simulink library "HEV_Electrical_Lib"  (R2019b)
settings: Solver=ode23t  StartTime=0.0  StopTime=10.0  MaxStep=1e-3  RelTol=1e-3
undefined symbols (not defined in the file): DiscIntNeverNeededParam, HEV_Param, magnitude, Ts
libraries: fl_lib x83, powerlib x61, nesl_utility x32, simulink_extras x8, simulink x6, electricdrivelib x4, HEV_Battery_Det_Lib x2, powerlib_extras x2, ee_lib x2, HEV_Battery_Lib x1
(part 2 of 4)

== system HEV_Electrical_Lib/System Level/Speed Sensor SyncGen ==
  MRRef : fl_lib/Mechanical/Rotational Elements/Mechanical Rotational Reference
  PS-Simulink Converter : nesl_utility/PS-Simulink Converter  PhysicalDomain=network_engine_domain  SubClassName=ps_output  LeftPortType=input  RightPortType=output  PseudoPeriodic=off  Frequencies=[]  Unit=rpm  AffineConversion=off
  Rotational Motion Sensor : fl_lib/Mechanical/Mechanical Sensors/Ideal Rotational Motion Sensor  offset=0 rad
  Sh : PMIOPort  Side=Left
  Sh1 : PMIOPort  Port=2  Side=Right
  tag scope: Gen_RPM_SYS=global
  wires:
  PS-Simulink Converter/1 -> [Gen_RPM_SYS]  "Gen_RPM"
  connections:
  Rotational Motion Sensor/RConn1 -- MRRef/LConn1
  PS-Simulink Converter/LConn1 -- Rotational Motion Sensor/RConn2
  Sh1/RConn1 -- Sh/RConn1 -- Rotational Motion Sensor/LConn1

== system HEV_Electrical_Lib/System Level/Speed Sensor SyncMot ==
  MRRef : fl_lib/Mechanical/Rotational Elements/Mechanical Rotational Reference
  PS-Simulink Converter : nesl_utility/PS-Simulink Converter  PhysicalDomain=network_engine_domain  SubClassName=ps_output  LeftPortType=input  RightPortType=output  PseudoPeriodic=off  Frequencies=[]  Unit=rpm  AffineConversion=off
  Rotational Motion Sensor : fl_lib/Mechanical/Mechanical Sensors/Ideal Rotational Motion Sensor  offset=0 rad
  Sh : PMIOPort  Side=Left
  Sh1 : PMIOPort  Port=2  Side=Right
  tag scope: Mot_RPM_SYS=global
  wires:
  PS-Simulink Converter/1 -> [Mot_RPM_SYS]  "Mot_RPM"
  connections:
  Rotational Motion Sensor/RConn1 -- MRRef/LConn1
  Sh1/RConn1 -- Rotational Motion Sensor/LConn1 -- Sh/RConn1
  PS-Simulink Converter/LConn1 -- Rotational Motion Sensor/RConn2

== system HEV_Electrical_Lib/System Level/Synchronous Generator & Drive ==
  note: Note that the generator can turn backwards - this happens when accelerating from rest. The
      | generator also acts as a starter for the engine. If the engine is running, then the generator
      | controller is used to manage battery charging using torque-control mode, otherwise the
      | generator controller controls generator speed.
  TReq : Inport
  GF : Subsystem
      mask Display: disp('GF')
  Inertia : fl_lib/Mechanical/Rotational Elements/Inertia  inertia=HEV_Param.Generator.Shaft_Inertia kg*m^2  w_specify=on  w_priority=High  w=0 rad/s  w_nominal_specify=off  w_nominal_unit=rad/s  w_nominal_value=1  t_specify=off  t_priority=High  t=0 N*m  t_nominal_specify=off  t_nominal_unit=N*m  t_nominal_value=1
  MRRef : fl_lib/Mechanical/Rotational Elements/Mechanical Rotational Reference
  PS Terminator : Subsystem
      mask Display:
      | plot([0 0.9],[0.5 0.5]);
      | plot([0.5 0.9],[0.3 0.3]);
      | plot([0.5 0.9],[0.7 0.7]);
      | plot([0.9 0.9],[0.7 0.3]);
  Power Sensor : Subsystem
      mask Display: disp('S')
  Power and Torque Sensor : Subsystem
      mask Display: disp('S')
  Servomotor : ee_lib/Electromechanical/Permanent Magnet/Simplified PMSM Drive  torque_speed_param=1  w_t=HEV_Param.Generator.TorqSpdLUT.SpeedRPM rpm  T_t=HEV_Param.Generator.TorqSpdLUT.TorqueNm N*m  torque_max=0.1 N*m  power_max=30 W  Tc=HEV_Param.Generator.TorqueControl_TimeConst s  losses_param=1  eff=90  w_eff=2000 rpm  T_eff=200 N*m  Piron=0 W  Pbase=HEV_Param.Generator.TorqIndep_Elec_Loss W  w_eff_vec=[-8000 -4000 0 4000 8000] rpm  T_eff_vec=[0 0.03 0.06 0.09] N*m  v_eff_vec=[100, 250, 400] V  losses_mat=[1.49 1.67 2.21 3.10; 0.42 0.69 1.14 2.03; 0.06 0.24 0.78 1.68; 0.42 0.69 1.14 2.03; 1.49 1.67 2.21 3.10] W  efficiency_mat=[95 95 95 95; 95 95 95 95; 95 95 95 95; 95 95 95 95; 95 95 95 95]  losses_mat_3D=ones(5, 4, 3) W  efficiency_mat_3D=95 * ones(5, 4, 3)  Res=HEV_Param.Generator.Series_Resistance Ohm  J=0 kg*m^2  lam=HEV_Param.Generator.Damping N*m/(rad/s)  speed0=0 rpm  faulted_specify=off  faulted_priority=None  faulted=0  faulted_nominal_specify=off  faulted_nominal_unit=1  faulted_nominal_value=1  alpha=3.93e-3 1/K  Tmeas=25 degC  Tmeas2=125 degC  losses_mat_T2=[1.49, 1.74, 2.49, 3.74; .42, .67, 1.42, 2.67; .06, .31, 1.06, 2.31; .42, .67, 1.42, 2.67; 1.49, 1.74, 2.49, 3.74] W  efficiency_mat_T2=[95, 95, 95, 95; 95, 95, 95, 95; 95, 95, 95, 95; 95, 95, 95, 95; 95, 95, 95, 95]  losses_mat_3D_T2=ones(5, 4, 3) W  efficiency_mat_3D_T2=95 * ones(5, 4, 3)  thermal_mass=100 J/K  initial_temperature=25 degC  fault_condition=1  fault_threshold=0.5
      settings: SourceProductName=Simscape Electrical  SourceProductBaseCode=PS  InternalSimscapePortConfiguration="{\"Bottom\":[],\"Left\":[{\"id\":\"Vp\",\"label\":\"+\",\"type\":\"foundation.electrical.electrical\"},{\"id\":\"Tr\",\"label\":\"Tr\",\"type\":\"input\"},{\"id\":\"R\",\"label\":\"R\",\"type\":\"foundation.mechanical.rotational.rotational\"}],\"Right\":[{\"id\":\"Vm\",\"label\":\"-\",\"type\":\"foundation.electrical.electrical\"},{\"id\":\"Omega\",\"label\":\"w\",\"type\":\"output\"},{\"id\":\"C\",\"label\":\"C\",\"type\":\"foundation.mechanical.rotational.rotational\"}],\"Top\":[]}"
  Vcc : PMIOPort  Side=Right
  Gnd : PMIOPort  Port=2  Side=Right
  Shaft : PMIOPort  Port=3  Side=Right
  wires:
  TReq/1 -> GF/1(In1)
  connections:
  MRRef/LConn1 -- Servomotor/RConn3
  Power and Torque Sensor/LConn1 -- Servomotor/LConn3
  PS Terminator/LConn1 -- Servomotor/RConn2
  GF/RConn1 -- Servomotor/LConn2
  Power Sensor/RConn1 -- Servomotor/LConn1
  Vcc/RConn1 -- Power Sensor/LConn1
  Gnd/RConn1 -- Servomotor/RConn1 -- Power Sensor/LConn2
  Power and Torque Sensor/RConn1 -- Inertia/LConn1 -- Shaft/RConn1

== system HEV_Electrical_Lib/System Level/Synchronous Motor & Drive ==
  TReq : Inport
  GF : Subsystem
      mask Display: disp('GF')
  Inertia : fl_lib/Mechanical/Rotational Elements/Inertia  inertia=HEV_Param.Motor.Shaft_Inertia kg*m^2  w_specify=on  w_priority=High  w=0 rad/s  w_nominal_specify=off  w_nominal_unit=rad/s  w_nominal_value=1  t_specify=off  t_priority=High  t=0 N*m  t_nominal_specify=off  t_nominal_unit=N*m  t_nominal_value=1
  MRRef : fl_lib/Mechanical/Rotational Elements/Mechanical Rotational Reference
  PS Terminator1 : Subsystem
      mask Display:
      | plot([0 0.9],[0.5 0.5]);
      | plot([0.5 0.9],[0.3 0.3]);
      | plot([0.5 0.9],[0.7 0.7]);
      | plot([0.9 0.9],[0.7 0.3]);
  Power Sensor : Subsystem
      mask Display: disp('S')
  Power and Torque Sensor : Subsystem
      mask Display: disp('S')
  Servomotor : ee_lib/Electromechanical/Permanent Magnet/Simplified PMSM Drive  torque_speed_param=1  w_t=HEV_Param.Motor.TorqSpdLUT.SpeedRPM rpm  T_t=HEV_Param.Motor.TorqSpdLUT.TorqueNm N*m  torque_max=0.1 N*m  power_max=30 W  Tc=HEV_Param.Motor.TorqueControl_TimeConst s  losses_param=1  eff=HEV_Param.Motor.Efficiency  w_eff=2000 rpm  T_eff=200 N*m  Piron=0 W  Pbase=0 W  w_eff_vec=[-8000 -4000 0 4000 8000] rpm  T_eff_vec=[0 0.03 0.06 0.09] N*m  v_eff_vec=[100, 250, 400] V  losses_mat=[1.49 1.67 2.21 3.10; 0.42 0.69 1.14 2.03; 0.06 0.24 0.78 1.68; 0.42 0.69 1.14 2.03; 1.49 1.67 2.21 3.10] W  efficiency_mat=[95 95 95 95; 95 95 95 95; 95 95 95 95; 95 95 95 95; 95 95 95 95]  losses_mat_3D=ones(5, 4, 3) W  efficiency_mat_3D=95 * ones(5, 4, 3)  Res=HEV_Param.Motor.Series_Resistance Ohm  J=0 kg*m^2  lam=HEV_Param.Motor.Damping N*m/(rad/s)  speed0=0 rpm  faulted_specify=off  faulted_priority=None  faulted=0  faulted_nominal_specify=off  faulted_nominal_unit=1  faulted_nominal_value=1  alpha=3.93e-3 1/K  Tmeas=25 degC  Tmeas2=125 degC  losses_mat_T2=[1.49, 1.74, 2.49, 3.74; .42, .67, 1.42, 2.67; .06, .31, 1.06, 2.31; .42, .67, 1.42, 2.67; 1.49, 1.74, 2.49, 3.74] W  efficiency_mat_T2=[95, 95, 95, 95; 95, 95, 95, 95; 95, 95, 95, 95; 95, 95, 95, 95; 95, 95, 95, 95]  losses_mat_3D_T2=ones(5, 4, 3) W  efficiency_mat_3D_T2=95 * ones(5, 4, 3)  thermal_mass=100 J/K  initial_temperature=25 degC  fault_condition=1  fault_threshold=0.5
      settings: SourceProductName=Simscape Electrical  SourceProductBaseCode=PS  InternalSimscapePortConfiguration="{\"Bottom\":[],\"Left\":[{\"id\":\"Vp\",\"label\":\"+\",\"type\":\"foundation.electrical.electrical\"},{\"id\":\"Tr\",\"label\":\"Tr\",\"type\":\"input\"},{\"id\":\"R\",\"label\":\"R\",\"type\":\"foundation.mechanical.rotational.rotational\"}],\"Right\":[{\"id\":\"Vm\",\"label\":\"-\",\"type\":\"foundation.electrical.electrical\"},{\"id\":\"Omega\",\"label\":\"w\",\"type\":\"output\"},{\"id\":\"C\",\"label\":\"C\",\"type\":\"foundation.mechanical.rotational.rotational\"}],\"Top\":[]}"
  Vcc : PMIOPort  Side=Right
  Gnd : PMIOPort  Port=2  Side=Right
  Shaft : PMIOPort  Port=3  Side=Right
  wires:
  TReq/1 -> GF/1(In1)
  connections:
  Servomotor/RConn3 -- MRRef/LConn1
  Power and Torque Sensor/LConn1 -- Servomotor/LConn3
  GF/RConn1 -- Servomotor/LConn2
  Power Sensor/RConn1 -- Servomotor/LConn1
  Vcc/RConn1 -- Power Sensor/LConn1
  Servomotor/RConn1 -- Gnd/RConn1 -- Power Sensor/LConn2
  PS Terminator1/LConn1 -- Servomotor/RConn2
  Inertia/LConn1 -- Power and Torque Sensor/RConn1 -- Shaft/RConn1

== system HEV_Electrical_Lib/System Level/Voltage Sensor ==
  PS-Simulink Converter : nesl_utility/PS-Simulink Converter  PhysicalDomain=network_engine_domain  SubClassName=ps_output  LeftPortType=input  RightPortType=output  PseudoPeriodic=off  Frequencies=[]  Unit=V  AffineConversion=off
  Voltage Sensor : fl_lib/Electrical/Electrical Sensors/Voltage Sensor
  + : PMIOPort  Side=Left
  - : PMIOPort  Port=2  Side=Right
  tag scope: DC_Bus_SYS=global
  wires:
  PS-Simulink Converter/1 -> [DC_Bus_SYS]
  connections:
  -/RConn1 -- Voltage Sensor/RConn2
  +/RConn1 -- Voltage Sensor/LConn1
  Voltage Sensor/RConn1 -- PS-Simulink Converter/LConn1

== system HEV_Electrical_Lib/Detailed/DC//DC Converter/PWM ==
  Ref. : Inport
  Data Type Conversion : DataTypeConversion  SaturateOnIntegerOverflow=on  RndMeth=Zero
  Data Type Conversion1 : DataTypeConversion  SaturateOnIntegerOverflow=on  RndMeth=Zero
  Mux : Mux  Inputs=2
  NOT : Logic  Operator=NOT  Inputs=1  AllPortsSameDT=off  OutDataTypeStr=uint(8)
  Rate Transition : RateTransition
  Relational Operator : RelationalOperator  Operator=>  RndMeth=Nearest
  Sawtooth generator : Subsystem
  Thermal Model : Subsystem
  Zero-Order Hold : ZeroOrderHold  SampleTime=Ts
  Pulses : Outport  VectorParamsAs1DForOutWhenUnconnected=off
  wires:
  NOT/1 -> Mux/2
  Rate Transition/1 -> Zero-Order Hold/1
  Relational Operator/1 -> Data Type Conversion/1
  Data Type Conversion/1 -> Mux/1, NOT/1
  Zero-Order Hold/1 -> Relational Operator/1
  Sawtooth generator/1(Out) -> Relational Operator/2
  Ref./1 -> Rate Transition/1, Thermal Model/1(IBus)
  Mux/1 -> Data Type Conversion1/1
  Data Type Conversion1/1 -> Pulses/1

== system HEV_Electrical_Lib/Detailed/DC//DC Converter/Voltage Controller ==
  Uref : Inport
  UBus : Inport  Port=2
  Clock1 : Clock
  Compare To Constant1 : simulink/Logic and Bit Operations/Compare To Constant  relop=>  const=0.01  OutDataTypeStr=uint8  ZeroCross=off
  Ctrl sat. : Saturate  UpperLimit=0.95  LowerLimit=-0.95
  Discrete-Time Integrator : DiscreteIntegrator  IntegratorMethod=Integration: Trapezoidal  SampleTime=Ts  LimitOutput=on  UpperSaturationLimit=1  LowerSaturationLimit=-1  ICPrevOutput=DiscIntNeverNeededParam  ICPrevScaledInput=DiscIntNeverNeededParam
  Integral gain : Gain  Gain=Ki  SaturateOnIntegerOverflow=on  OutDataTypeStr=Inherit: Same as input  ParamDataTypeStr=Inherit: Same as input
  Product1 : Product  RndMeth=Zero
  Proportional gain : Gain  Gain=Kp  SaturateOnIntegerOverflow=on  OutDataTypeStr=Inherit: Same as input  ParamDataTypeStr=Inherit: Same as input
  Sum1 : Sum  Inputs=+-  SaturateOnIntegerOverflow=on  InputSameDT=on  OutDataTypeStr=Inherit: Same as first input
  Sum2 : Sum  SaturateOnIntegerOverflow=on  InputSameDT=on  OutDataTypeStr=Inherit: Same as first input
  Transfer Fcn : TransferFcn  Denominator=[.0001 1]
  Zero-Order Hold1 : ZeroOrderHold  SampleTime=Ts
  Ec : Outport  InitialOutput=0  VectorParamsAs1DForOutWhenUnconnected=off
  wires:
  Sum2/1 -> Ctrl sat./1
  Discrete-Time Integrator/1 -> Sum2/2
  UBus/1 -> Zero-Order Hold1/1
  Integral gain/1 -> Discrete-Time Integrator/1
  Proportional gain/1 -> Sum2/1
  Ctrl sat./1 -> Ec/1
  Sum1/1 -> Product1/1
  Clock1/1 -> Compare To Constant1/1
  Compare To Constant1/1 -> Product1/2
  Product1/1 -> Integral gain/1, Proportional gain/1
  Zero-Order Hold1/1 -> Transfer Fcn/1
  Transfer Fcn/1 -> Sum1/1
  Uref/1 -> Sum1/2

== system HEV_Electrical_Lib/Detailed/Synchronous Generator & Drive/GF ==
  In1 : Inport
  Out1 : Outport  VectorParamsAs1DForOutWhenUnconnected=off
  tag scope: Gen_TReq_SYS=global
  wires:
  In1/1 -> Out1/1, [Gen_TReq_SYS]

== system HEV_Electrical_Lib/Detailed/Synchronous Generator & Drive/Mux ==
  gates : Inport
  m : Inport  Port=2
  Terminator : Terminator
  g : Outport  VectorParamsAs1DForOutWhenUnconnected=off
  wires:
  gates/1 -> g/1
  m/1 -> Terminator/1

== system HEV_Electrical_Lib/Detailed/Synchronous Generator & Drive/Subsystem ==
  In : Inport
  "+ -> -1" : Gain  Gain=30/pi
  Bus Selector : BusSelector  OutputSignals=Stator current is_a (A),Rotor speed wm (rad/s),Electromagnetic torque Te (N*m)
  Mux1 : Mux  Inputs=2
  Mux2 : Mux  Inputs=3
  Out : Outport  VectorParamsAs1DForOutWhenUnconnected=off
  tag scope: GeneratorDrive=global
  wires:
  In/1 -> Bus Selector/1, Out/1
  "+ -> -1"/1 -> Mux2/2
  [Gen_TReq_SYS] -> Mux1/2
  Bus Selector/2 -> "+ -> -1"/1  "<Rotor speed wm (rad/s)>"
  Bus Selector/3 -> Mux1/1  "<Electromagnetic torque Te (N*m)>"
  Mux1/1 -> Mux2/3
  Bus Selector/1 -> Mux2/1  "<Stator current is_a (A)>"
  Mux2/1 -> [GeneratorDrive]

== system HEV_Electrical_Lib/Detailed/Synchronous Generator & Drive/Subsystem1 ==
  Sig : Inport
  Bus Selector : BusSelector  OutputSignals=Electromagnetic torque Te (N*m)
  Ideal Rotational Motion Sensor : fl_lib/Mechanical/Mechanical Sensors/Ideal Rotational Motion Sensor  offset=0 rad
  Ideal Torque Source : fl_lib/Mechanical/Mechanical Sources/Ideal Torque Source
  Mechanical Rotational Reference : fl_lib/Mechanical/Rotational Elements/Mechanical Rotational Reference
  Mechanical Rotational Reference1 : fl_lib/Mechanical/Rotational Elements/Mechanical Rotational Reference
  PS-Simulink Converter : nesl_utility/PS-Simulink Converter  PhysicalDomain=network_engine_domain  SubClassName=ps_output  LeftPortType=input  RightPortType=output  PseudoPeriodic=off  Frequencies=[]  Unit=rad/s  AffineConversion=off
  Simulink-PS Converter : nesl_utility/Simulink-PS Converter  PhysicalDomain=network_engine_domain  SubClassName=ps_input  LeftPortType=input  RightPortType=output  PseudoPeriodic=off  Frequencies=[]  NoiseDistribution=none  NoiseParameters=[]  Unit=1  AffineConversion=off  FilteringAndDerivatives=zero  SimscapeFilterOrder=1  InputFilterTimeConstant=0.005  UdotUserProvided=0
  Sh : PMIOPort  Side=Right
  Spd : Outport  VectorParamsAs1DForOutWhenUnconnected=off
  wires:
  Bus Selector/1 -> Simulink-PS Converter/1  "<Electromagnetic torque Te (N*m)>"
  Sig/1 -> Bus Selector/1
  PS-Simulink Converter/1 -> Spd/1
  connections:
  Mechanical Rotational Reference/LConn1 -- Ideal Rotational Motion Sensor/RConn1
  Mechanical Rotational Reference1/LConn1 -- Ideal Torque Source/RConn2
  Ideal Torque Source/LConn1 -- Sh/RConn1 -- Ideal Rotational Motion Sensor/LConn1
  PS-Simulink Converter/LConn1 -- Ideal Rotational Motion Sensor/RConn2
  Simulink-PS Converter/RConn1 -- Ideal Torque Source/RConn1

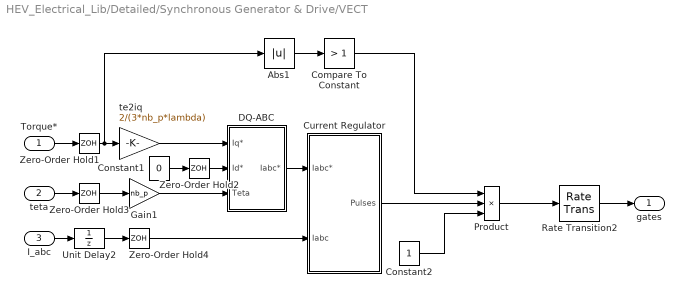
== system HEV_Electrical_Lib/Detailed/Synchronous Generator & Drive/VECT ==
  Torque* : Inport
  teta : Inport  Port=2
  I_abc : Inport  Port=3
  Abs1 : Abs
  Compare To Constant : simulink/Logic and Bit Operations/Compare To Constant  relop=>  const=1  OutDataTypeStr=uint8
  Constant1 : Constant  Value=0
  Constant2 : Constant
  Current Regulator : Subsystem
  DQ-ABC : Subsystem
  Gain1 : Gain  Gain=nb_p  SaturateOnIntegerOverflow=on  OutDataTypeStr=Inherit: Same as input  ParamDataTypeStr=Inherit: Same as input
  Product : Product  Inputs=3  RndMeth=Zero
  Rate Transition2 : RateTransition
  Unit Delay2 : UnitDelay  SampleTime=-1  HasFrameUpgradeWarning=on
  Zero-Order Hold{1..4} (4 alike) : ZeroOrderHold  SampleTime=Ts_vect
  te2iq : Gain  Gain=2/(3*nb_p*lambda)  SaturateOnIntegerOverflow=on  OutDataTypeStr=Inherit: Same as input  ParamDataTypeStr=Inherit: Same as input
  gates : Outport  VectorParamsAs1DForOutWhenUnconnected=off
  wires:
  Compare To Constant/1 -> Product/1
  Abs1/1 -> Compare To Constant/1
  Constant2/1 -> Product/3
  I_abc/1 -> Unit Delay2/1
  DQ-ABC/1(Iabc*) -> Current Regulator/1(Iabc*)
  Gain1/1 -> DQ-ABC/3(Teta)
  Constant1/1 -> Zero-Order Hold2/1
  Torque*/1 -> Zero-Order Hold1/1
  Zero-Order Hold3/1 -> Gain1/1
  teta/1 -> Zero-Order Hold3/1
  Current Regulator/1(Pulses) -> Product/2
  Zero-Order Hold1/1 -> Abs1/1, te2iq/1
  Zero-Order Hold4/1 -> Current Regulator/2(Iabc)
  Zero-Order Hold2/1 -> DQ-ABC/2("Id* ")
  Rate Transition2/1 -> gates/1
  Product/1 -> Rate Transition2/1
  te2iq/1 -> DQ-ABC/1("Iq* ")
  Unit Delay2/1 -> Zero-Order Hold4/1

== system HEV_Electrical_Lib/Detailed/Synchronous Motor & Drive/GF ==
  In1 : Inport
  Out1 : Outport  VectorParamsAs1DForOutWhenUnconnected=off
  tag scope: Mot_TReq_SYS=global
  wires:
  In1/1 -> Out1/1, [Mot_TReq_SYS]

== system HEV_Electrical_Lib/Detailed/Synchronous Motor & Drive/Mux ==
  gates : Inport
  m : Inport  Port=2
  Terminator : Terminator
  g : Outport  VectorParamsAs1DForOutWhenUnconnected=off
  wires:
  m/1 -> Terminator/1
  gates/1 -> g/1

== system HEV_Electrical_Lib/Detailed/Synchronous Motor & Drive/Subsystem ==
  In : Inport
  "+ -> -1" : Gain  Gain=30/pi
  Bus Selector : BusSelector  OutputSignals=Stator current is_a (A),Rotor speed wm (rad/s),Electromagnetic torque Te (N*m)
  Mux1 : Mux  Inputs=2
  Mux2 : Mux  Inputs=3
  Out : Outport  VectorParamsAs1DForOutWhenUnconnected=off
  tag scope: MotorDrive=global
  wires:
  In/1 -> Bus Selector/1, Out/1
  "+ -> -1"/1 -> Mux2/2
  [Mot_TReq_SYS] -> Mux1/2
  Bus Selector/2 -> "+ -> -1"/1  "<Rotor speed wm (rad/s)>"
  Bus Selector/3 -> Mux1/1  "<Electromagnetic torque Te (N*m)>"
  Mux1/1 -> Mux2/3
  Bus Selector/1 -> Mux2/1  "<Stator current is_a (A)>"
  Mux2/1 -> [MotorDrive]

== system HEV_Electrical_Lib/Detailed/Synchronous Motor & Drive/Subsystem1 ==
  Sig : Inport
  Bus Selector : BusSelector  OutputSignals=Electromagnetic torque Te (N*m)
  Ideal Rotational Motion Sensor : fl_lib/Mechanical/Mechanical Sensors/Ideal Rotational Motion Sensor  offset=0 rad
  Ideal Torque Source : fl_lib/Mechanical/Mechanical Sources/Ideal Torque Source
  Mechanical Rotational Reference : fl_lib/Mechanical/Rotational Elements/Mechanical Rotational Reference
  Mechanical Rotational Reference1 : fl_lib/Mechanical/Rotational Elements/Mechanical Rotational Reference
  PS-Simulink Converter : nesl_utility/PS-Simulink Converter  PhysicalDomain=network_engine_domain  SubClassName=ps_output  LeftPortType=input  RightPortType=output  PseudoPeriodic=off  Frequencies=[]  Unit=rad/s  AffineConversion=off
  Simulink-PS Converter : nesl_utility/Simulink-PS Converter  PhysicalDomain=network_engine_domain  SubClassName=ps_input  LeftPortType=input  RightPortType=output  PseudoPeriodic=off  Frequencies=[]  NoiseDistribution=none  NoiseParameters=[]  Unit=1  AffineConversion=off  FilteringAndDerivatives=zero  SimscapeFilterOrder=1  InputFilterTimeConstant=0.005  UdotUserProvided=0
  Sh : PMIOPort  Side=Right
  Spd : Outport  VectorParamsAs1DForOutWhenUnconnected=off
  wires:
  PS-Simulink Converter/1 -> Spd/1
  Sig/1 -> Bus Selector/1
  Bus Selector/1 -> Simulink-PS Converter/1  "<Electromagnetic torque Te (N*m)>"
  connections:
  Simulink-PS Converter/RConn1 -- Ideal Torque Source/RConn1
  PS-Simulink Converter/LConn1 -- Ideal Rotational Motion Sensor/RConn2
  Ideal Rotational Motion Sensor/LConn1 -- Sh/RConn1 -- Ideal Torque Source/LConn1
  Mechanical Rotational Reference1/LConn1 -- Ideal Torque Source/RConn2
  Mechanical Rotational Reference/LConn1 -- Ideal Rotational Motion Sensor/RConn1

== system HEV_Electrical_Lib/Detailed/Synchronous Motor & Drive/Torque limitation ==
  N rad/s : Inport
  Torque : Inport  Port=2
  Abs1 : Abs  SaturateOnIntegerOverflow=on
  Gain : Gain  Gain=-1
  Saturation Dynamic : simulink/Discontinuities/Saturation Dynamic  OutMin=[]  OutMax=[]  OutDataTypeStr=Inherit: Same as second input  OutDataType=sfix(16)  OutScaling=2^-10  DoSatur=off
  Torque vs speed profile : Lookup  InputValues=[0 1200 2000 3000 4000 5000 6000]*pi/30  Table=[400 400 225 150 100 80 70]
  torque : Outport  VectorParamsAs1DForOutWhenUnconnected=off
  wires:
  Gain/1 -> Saturation Dynamic/3
  Torque/1 -> Saturation Dynamic/2
  Saturation Dynamic/1 -> torque/1
  Torque vs speed profile/1 -> Gain/1, Saturation Dynamic/1
  Abs1/1 -> Torque vs speed profile/1
  N rad/s/1 -> Abs1/1

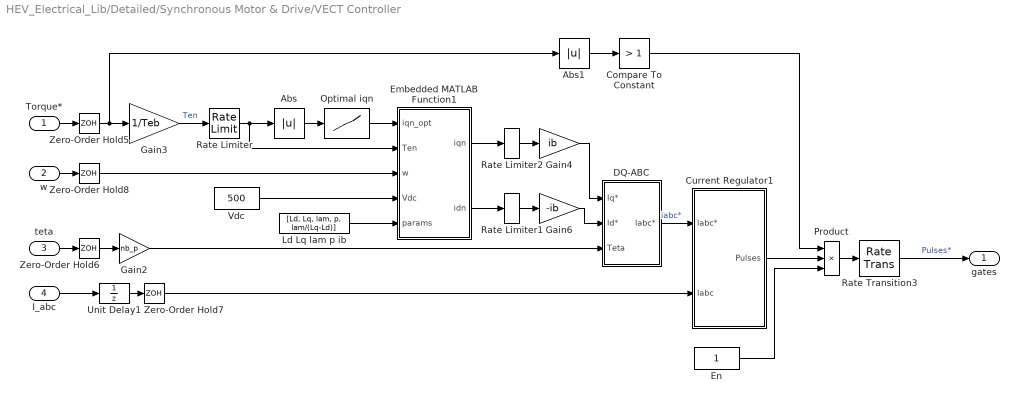
== system HEV_Electrical_Lib/Detailed/Synchronous Motor & Drive/VECT Controller ==
  Torque* : Inport
  w : Inport  Port=2
  teta : Inport  Port=3
  I_abc : Inport  Port=4
  Abs : Abs
  Abs1 : Abs
  Compare To Constant : simulink/Logic and Bit Operations/Compare To Constant  relop=>  const=1  OutDataTypeStr=uint8
  Current Regulator1 : Subsystem
  DQ-ABC : Subsystem
  Embedded MATLAB Function1 : MATLAB Function  TreatAsAtomicUnit=on  SystemSampleTime=Ts_vect
  En : Constant
  Gain2 : Gain  Gain=nb_p  SaturateOnIntegerOverflow=on  OutDataTypeStr=Inherit: Same as input  ParamDataTypeStr=Inherit: Same as input
  Gain3 : Gain  Gain=1/Teb  SaturateOnIntegerOverflow=on  OutDataTypeStr=Inherit: Same as input  ParamDataTypeStr=Inherit: Same as input
  Gain4 : Gain  Gain=ib  SaturateOnIntegerOverflow=on  OutDataTypeStr=Inherit: Same as input  ParamDataTypeStr=Inherit: Same as input
  Gain6 : Gain  Gain=-ib  SaturateOnIntegerOverflow=on  OutDataTypeStr=Inherit: Same as input  ParamDataTypeStr=Inherit: Same as input
  Ld Lq lam p ib : Constant  Value=[Ld, Lq, lam, p, lam/(Lq-Ld)]
  Optimal iqn : Lookup  InputValues=ten  Table=iqn
  Product : Product  Inputs=3  RndMeth=Zero
  Rate Limiter : RateLimiter  RisingSlewLimit=10  FallingSlewLimit=-10  LinearizeAsGain=off
  Rate Limiter1 : RateLimiter  RisingSlewLimit=100  FallingSlewLimit=-100  SampleTimeMode=inherited
  Rate Limiter2 : RateLimiter  RisingSlewLimit=100  FallingSlewLimit=-100  SampleTimeMode=inherited
  Rate Transition3 : RateTransition
  Unit Delay1 : UnitDelay  SampleTime=-1  HasFrameUpgradeWarning=on
  Vdc : Constant  Value=500
  Zero-Order Hold{5..8} (4 alike) : ZeroOrderHold  SampleTime=Ts_vect
  gates : Outport  VectorParamsAs1DForOutWhenUnconnected=off
  wires:
  Abs1/1 -> Compare To Constant/1
  Compare To Constant/1 -> Product/1
  En/1 -> Product/3
  Current Regulator1/1(Pulses) -> Product/2
  Unit Delay1/1 -> Zero-Order Hold7/1
  Zero-Order Hold7/1 -> Current Regulator1/2(Iabc)
  teta/1 -> Zero-Order Hold6/1
  Zero-Order Hold6/1 -> Gain2/1
  Gain2/1 -> DQ-ABC/3(Teta)
  DQ-ABC/1(Iabc*) -> Current Regulator1/1(Iabc*)  "iabc*"
  I_abc/1 -> Unit Delay1/1
  Torque*/1 -> Zero-Order Hold5/1
  Gain4/1 -> DQ-ABC/1("Iq* ")
  Gain6/1 -> DQ-ABC/2("Id* ")
  Zero-Order Hold5/1 -> Abs1/1, Gain3/1
  w/1 -> Zero-Order Hold8/1
  Embedded MATLAB Function1/2(idn) -> Rate Limiter1/1
  Gain3/1 -> Rate Limiter/1  "Ten"
  Zero-Order Hold8/1 -> Embedded MATLAB Function1/3(w)
  Ld Lq lam p ib/1 -> Embedded MATLAB Function1/5(params)
  Embedded MATLAB Function1/1(iqn) -> Rate Limiter2/1
  Optimal iqn/1 -> Embedded MATLAB Function1/1(iqn_opt)
  Abs/1 -> Optimal iqn/1
  Vdc/1 -> Embedded MATLAB Function1/4(Vdc)
  Rate Transition3/1 -> gates/1  "Pulses*"
  Product/1 -> Rate Transition3/1
  Rate Limiter2/1 -> Gain4/1
  Rate Limiter1/1 -> Gain6/1
  Rate Limiter/1 -> Abs/1, Embedded MATLAB Function1/2(Ten)

== system HEV_Electrical_Lib/Mean Value/DC//DC Converter/Boost Converter Average-Values ==
  Duty Cycle : Inport
  Average-value armature voltage : Fcn  Expr=u(1)*u(2)
  Average-value source current : Fcn  Expr=u(1)*u(2)
  Controlled Current Source : powerlib/Electrical Sources/Controlled Current Source  Initialize=on  Source_Type=AC  Amplitude=0  Phase=0  Frequency=0  Measurements=None
      settings: SourceProductName=Simscape Electrical
  Controlled Voltage Source : powerlib/Electrical Sources/Controlled Voltage Source  Initialize=on  Source_Type=AC  Amplitude=0  Phase=0  Frequency=0  Measurements=None
      settings: SourceProductName=Simscape Electrical
  Current Measurement : powerlib/Measurements/Current Measurement  Tag=PoWeRsYsTeMmEaSuReMeNt  PhasorSimulation=off  OutputType=Magnitude  PSBequivalent=0
      settings: SourceProductName=Simscape Electrical
  Mux : Mux  Inputs=2
  Mux1 : Mux  Inputs=2
  Selector : Selector  InputPortWidth=2  IndexOptions=Index vector (dialog)  Indices=[1]  OutputSizes=1
  Thermal Model : Subsystem
  Unit Delay : UnitDelay  SampleTime=Ts  HasFrameUpgradeWarning=on
  Unit Delay1 : UnitDelay  SampleTime=Ts  HasFrameUpgradeWarning=on
  Voltage Measurement1 : powerlib/Measurements/Voltage Measurement  Tag=PoWeRsYsTeMmEaSuReMeNt  PhasorSimulation=off  OutputType=Magnitude  PSBequivalent=0
      settings: SourceProductName=Simscape Electrical
  A : PMIOPort  Side=Right
  + : PMIOPort  Port=2  Side=Left
  - : PMIOPort  Port=3  Side=Left
  wires:
  Unit Delay/1 -> Controlled Voltage Source/1
  Average-value armature voltage/1 -> Unit Delay/1
  Mux/1 -> Average-value armature voltage/1
  Voltage Measurement1/1 -> Mux/2
  Duty Cycle/1 -> Selector/1
  Mux1/1 -> Average-value source current/1
  Current Measurement/1 -> Mux1/2
  Average-value source current/1 -> Unit Delay1/1
  Unit Delay1/1 -> Controlled Current Source/1, Thermal Model/1(IBus)
  Selector/1 -> Mux/1, Mux1/1
  connections:
  Voltage Measurement1/LConn2 -- Controlled Current Source/RConn1 -- -/RConn1 -- Controlled Voltage Source/LConn1
  Controlled Current Source/LConn1 -- Voltage Measurement1/LConn1 -- +/RConn1
  Controlled Voltage Source/RConn1 -- Current Measurement/LConn1
  A/RConn1 -- Current Measurement/RConn1

== system HEV_Electrical_Lib/Mean Value/DC//DC Converter/Current controller DISCRETE3 ==
  Uref : Inport
  UBus : Inport  Port=2
  Clock1 : Clock
  Compare To Constant1 : simulink/Logic and Bit Operations/Compare To Constant  relop=>  const=0.01  OutDataTypeStr=uint8  ZeroCross=off
  Ctrl sat. : Saturate  UpperLimit=0.95  LowerLimit=-0.95
  Discrete-Time Integrator : DiscreteIntegrator  IntegratorMethod=Integration: Trapezoidal  SampleTime=Ts  LimitOutput=on  UpperSaturationLimit=1  LowerSaturationLimit=-1  ICPrevOutput=DiscIntNeverNeededParam  ICPrevScaledInput=DiscIntNeverNeededParam
  Integral gain : Gain  Gain=Ki  SaturateOnIntegerOverflow=on  OutDataTypeStr=Inherit: Same as input  ParamDataTypeStr=Inherit: Same as input
  Product1 : Product  RndMeth=Zero
  Proportional gain : Gain  Gain=Kp  SaturateOnIntegerOverflow=on  OutDataTypeStr=Inherit: Same as input  ParamDataTypeStr=Inherit: Same as input
  Sum1 : Sum  Inputs=+-  SaturateOnIntegerOverflow=on  InputSameDT=on  OutDataTypeStr=Inherit: Same as first input
  Sum2 : Sum  SaturateOnIntegerOverflow=on  InputSameDT=on  OutDataTypeStr=Inherit: Same as first input
  Transfer Fcn : TransferFcn  Denominator=[.0001 1]
  Zero-Order Hold1 : ZeroOrderHold  SampleTime=Ts
  Ec : Outport  InitialOutput=0  VectorParamsAs1DForOutWhenUnconnected=off
  wires:
  Sum2/1 -> Ctrl sat./1
  Discrete-Time Integrator/1 -> Sum2/2
  UBus/1 -> Zero-Order Hold1/1
  Integral gain/1 -> Discrete-Time Integrator/1
  Proportional gain/1 -> Sum2/1
  Ctrl sat./1 -> Ec/1
  Sum1/1 -> Product1/1
  Clock1/1 -> Compare To Constant1/1
  Compare To Constant1/1 -> Product1/2
  Product1/1 -> Integral gain/1, Proportional gain/1
  Zero-Order Hold1/1 -> Transfer Fcn/1
  Transfer Fcn/1 -> Sum1/1
  Uref/1 -> Sum1/2

== system HEV_Electrical_Lib/Mean Value/DC//DC Converter/Duty Cycles ==
  Ec : Inport
  Add : Sum  Inputs=+-
  Bus Creator2 : BusCreator  Inputs=2
  Constant : Constant
  Duty Cycle : Fcn  Expr=0.5*(u[1]+1)
  Unit Delay2 : UnitDelay  InitialCondition=.5  SampleTime=Ts  HasFrameUpgradeWarning=on
  dc : Outport  VectorParamsAs1DForOutWhenUnconnected=off
  wires:
  Bus Creator2/1 -> Unit Delay2/1
  Ec/1 -> Duty Cycle/1
  Constant/1 -> Add/1
  Add/1 -> Bus Creator2/2  "IGBT 2"
  Duty Cycle/1 -> Bus Creator2/1, Add/2  "IGBT I"
  Unit Delay2/1 -> dc/1

== system HEV_Electrical_Lib/Mean Value/Synchronous Generator & Drive/GF ==
  In1 : Inport
  Out1 : Outport  VectorParamsAs1DForOutWhenUnconnected=off
  tag scope: Gen_TReq_SYS=global
  wires:
  In1/1 -> Out1/1, [Gen_TReq_SYS]

== system HEV_Electrical_Lib/Mean Value/Synchronous Generator & Drive/Mux ==
  sig* : Inport
  m : Inport  Port=2
  Bus Creator : BusCreator  Inputs=2
  Ctrl : Outport  VectorParamsAs1DForOutWhenUnconnected=off
  wires:
  Bus Creator/1 -> Ctrl/1
  sig*/1 -> Bus Creator/1  "Signals*"
  m/1 -> Bus Creator/2  "m"

== system HEV_Electrical_Lib/Mean Value/Synchronous Generator & Drive/Subsystem ==
  In : Inport
  "+ -> -1" : Gain  Gain=30/pi
  Bus Selector : BusSelector  OutputSignals=Stator current is_a (A),Rotor speed wm (rad/s),Electromagnetic torque Te (N*m)
  Mux1 : Mux  Inputs=2
  Mux2 : Mux  Inputs=3
  Out : Outport  VectorParamsAs1DForOutWhenUnconnected=off
  tag scope: GeneratorDrive=global
  wires:
  In/1 -> Bus Selector/1, Out/1
  "+ -> -1"/1 -> Mux2/2
  [Gen_TReq_SYS] -> Mux1/2
  Bus Selector/2 -> "+ -> -1"/1  "<Rotor speed wm (rad/s)>"
  Bus Selector/3 -> Mux1/1  "<Electromagnetic torque Te (N*m)>"
  Mux1/1 -> Mux2/3
  Bus Selector/1 -> Mux2/1  "<Stator current is_a (A)>"
  Mux2/1 -> [GeneratorDrive]

== system HEV_Electrical_Lib/Mean Value/Synchronous Generator & Drive/Subsystem1 ==
  Sig : Inport
  Bus Selector : BusSelector  OutputSignals=Electromagnetic torque Te (N*m)
  Ideal Rotational Motion Sensor : fl_lib/Mechanical/Mechanical Sensors/Ideal Rotational Motion Sensor  offset=0 rad
  Ideal Torque Source : fl_lib/Mechanical/Mechanical Sources/Ideal Torque Source
  Mechanical Rotational Reference : fl_lib/Mechanical/Rotational Elements/Mechanical Rotational Reference
  Mechanical Rotational Reference1 : fl_lib/Mechanical/Rotational Elements/Mechanical Rotational Reference
  PS-Simulink Converter : nesl_utility/PS-Simulink Converter  PhysicalDomain=network_engine_domain  SubClassName=ps_output  LeftPortType=input  RightPortType=output  PseudoPeriodic=off  Frequencies=[]  Unit=rad/s  AffineConversion=off
  Simulink-PS Converter : nesl_utility/Simulink-PS Converter  PhysicalDomain=network_engine_domain  SubClassName=ps_input  LeftPortType=input  RightPortType=output  PseudoPeriodic=off  Frequencies=[]  NoiseDistribution=none  NoiseParameters=[]  Unit=1  AffineConversion=off  FilteringAndDerivatives=zero  SimscapeFilterOrder=1  InputFilterTimeConstant=0.005  UdotUserProvided=0
  Sh : PMIOPort  Side=Right
  Spd : Outport  VectorParamsAs1DForOutWhenUnconnected=off
  wires:
  PS-Simulink Converter/1 -> Spd/1
  Sig/1 -> Bus Selector/1
  Bus Selector/1 -> Simulink-PS Converter/1  "<Electromagnetic torque Te (N*m)>"
  connections:
  Simulink-PS Converter/RConn1 -- Ideal Torque Source/RConn1
  PS-Simulink Converter/LConn1 -- Ideal Rotational Motion Sensor/RConn2
  Ideal Rotational Motion Sensor/LConn1 -- Sh/RConn1 -- Ideal Torque Source/LConn1
  Mechanical Rotational Reference1/LConn1 -- Ideal Torque Source/RConn2
  Mechanical Rotational Reference/LConn1 -- Ideal Rotational Motion Sensor/RConn1

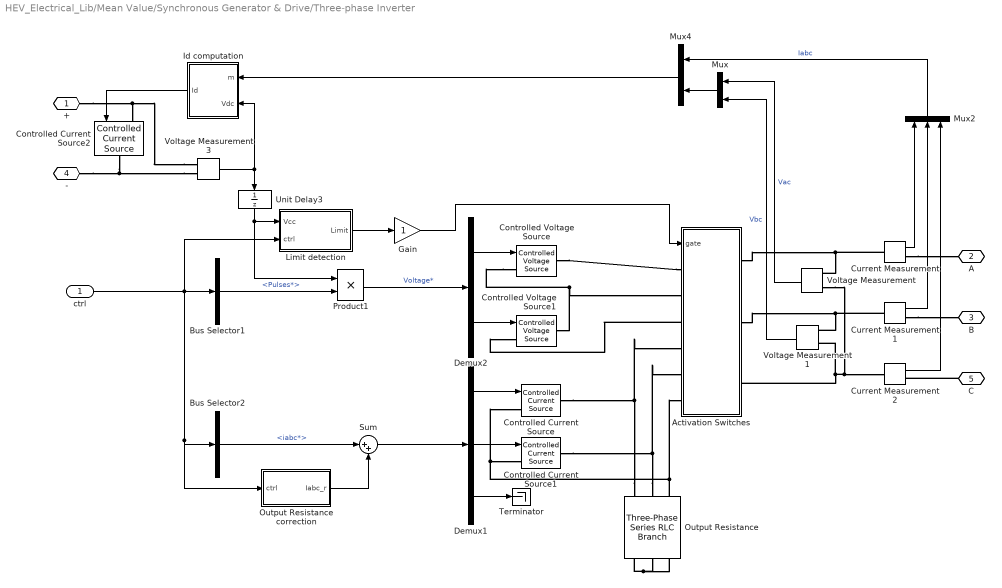
== system HEV_Electrical_Lib/Mean Value/Synchronous Generator & Drive/Three-phase Inverter ==
  ctrl : Inport
  Activation Switches : Subsystem
  Bus Selector1 : BusSelector  OutputSignals=Signals*.Pulses*
  Bus Selector2 : BusSelector  OutputSignals=Signals*.iabc*
  Controlled Current Source : powerlib/Electrical Sources/Controlled Current Source  Initialize=on  Source_Type=AC  Amplitude=0  Phase=0  Frequency=0  Measurements=None
      settings: SourceProductName=Simscape Electrical
  Controlled Current Source1 : powerlib/Electrical Sources/Controlled Current Source  Initialize=on  Source_Type=AC  Amplitude=0  Phase=0  Frequency=0  Measurements=None
      settings: SourceProductName=Simscape Electrical
  Controlled Current Source2 : powerlib/Electrical Sources/Controlled Current Source  Initialize=on  Source_Type=AC  Amplitude=0  Phase=0  Frequency=0  Measurements=None
      settings: SourceProductName=Simscape Electrical
  Controlled Voltage Source : powerlib/Electrical Sources/Controlled Voltage Source  Initialize=on  Source_Type=AC  Amplitude=0  Phase=0  Frequency=0  Measurements=None
      settings: SourceProductName=Simscape Electrical
  Controlled Voltage Source1 : powerlib/Electrical Sources/Controlled Voltage Source  Initialize=on  Source_Type=AC  Amplitude=0  Phase=0  Frequency=0  Measurements=None
      settings: SourceProductName=Simscape Electrical
  Current Measurement : powerlib/Measurements/Current Measurement  PhasorSimulation=off  OutputType=Complex  PSBequivalent=0
      settings: SourceProductName=Simscape Electrical
  Current Measurement1 : powerlib/Measurements/Current Measurement  PhasorSimulation=off  OutputType=Complex  PSBequivalent=0
      settings: SourceProductName=Simscape Electrical
  Current Measurement2 : powerlib/Measurements/Current Measurement  PhasorSimulation=off  OutputType=Complex  PSBequivalent=0
      settings: SourceProductName=Simscape Electrical
  Demux1 : Demux  Outputs=3
  Demux2 : Demux  Outputs=2
  Gain : Gain
  Id computation : Subsystem
  Limit detection : Subsystem
  Mux : Mux  Inputs=2
  Mux2 : Mux  Inputs=3
  Mux4 : Mux  Inputs=2
  Output Resistance : powerlib/Elements/Three-Phase Series RLC Branch  LConnTagsString=A|B|C  RConnTagsString=A|B|C  BranchType=R  Resistance=100*Resistance  Inductance=1e-3  Capacitance=1e-6  Measurements=Branch voltages and currents
      settings: SourceProductName=Simscape Electrical
  Output Resistance correction : Subsystem
  Product1 : Product  RndMeth=Zero
  Sum : Sum  Inputs=|++
  Terminator : Terminator
  Unit Delay3 : UnitDelay  SampleTime=Ts  HasFrameUpgradeWarning=on
  Voltage Measurement : powerlib/Measurements/Voltage Measurement  PhasorSimulation=off  OutputType=Complex  PSBequivalent=0
      settings: SourceProductName=Simscape Electrical
  Voltage Measurement1 : powerlib/Measurements/Voltage Measurement  PhasorSimulation=off  OutputType=Complex  PSBequivalent=0
      settings: SourceProductName=Simscape Electrical
  Voltage Measurement3 : powerlib/Measurements/Voltage Measurement  PhasorSimulation=off  OutputType=Complex  PSBequivalent=0
      settings: SourceProductName=Simscape Electrical
  + : PMIOPort  Side=Right
  A : PMIOPort  Port=2  Side=Left
  B : PMIOPort  Port=3  Side=Left
  - : PMIOPort  Port=4  Side=Right
  C : PMIOPort  Port=5  Side=Left
  wires:
  Current Measurement/1 -> Mux2/1
  Current Measurement1/1 -> Mux2/2
  Voltage Measurement/1 -> Mux/1  "Vac"
  Voltage Measurement1/1 -> Mux/2  "Vbc"
  Mux/1 -> Mux4/2
  Current Measurement2/1 -> Mux2/3
  Mux4/1 -> Id computation/1(m)
  Mux2/1 -> Mux4/1  "Iabc"
  Id computation/1(Id) -> Controlled Current Source2/1
  Voltage Measurement3/1 -> Unit Delay3/1, Id computation/2(Vdc)
  Bus Selector1/1 -> Product1/2  "<Pulses*>"
  Demux1/1 -> Controlled Current Source/1
  Demux1/2 -> Controlled Current Source1/1
  Demux1/3 -> Terminator/1
  Demux2/2 -> Controlled Voltage Source1/1
  Demux2/1 -> Controlled Voltage Source/1
  Bus Selector2/1 -> Sum/1  "<iabc*>"
  Limit detection/1(Limit) -> Gain/1
  Sum/1 -> Demux1/1
  Unit Delay3/1 -> Product1/1, Limit detection/1(Vcc)
  ctrl/1 -> Bus Selector1/1, Limit detection/2(ctrl), Bus Selector2/1, Output Resistance correction/1(ctrl)
  Product1/1 -> Demux2/1  "Voltage*"
  Output Resistance correction/1("Iabc_r ") -> Sum/2
  Gain/1 -> Activation Switches/1(gate)
  connections:
  Voltage Measurement3/LConn1 -- Controlled Current Source2/LConn1 -- +/RConn1
  Voltage Measurement3/LConn2 -- Controlled Current Source2/RConn1 -- -/RConn1
  Activation Switches/LConn6 -- Controlled Current Source/LConn1 -- Controlled Current Source1/LConn1 -- Output Resistance/LConn3
  Output Resistance/RConn3 -- Output Resistance/RConn2 -- Output Resistance/RConn1
  Voltage Measurement/LConn1 -- Activation Switches/RConn1 -- Current Measurement/LConn1
  Output Resistance/LConn1 -- Activation Switches/LConn4 -- Controlled Current Source/RConn1
  Output Resistance/LConn2 -- Activation Switches/LConn5 -- Controlled Current Source1/RConn1
  Voltage Measurement/LConn2 -- Activation Switches/RConn3 -- Voltage Measurement1/LConn2 -- Current Measurement2/LConn1
  Controlled Voltage Source/LConn1 -- Activation Switches/LConn2 -- Controlled Voltage Source1/RConn1
  Voltage Measurement1/LConn1 -- Activation Switches/RConn2 -- Current Measurement1/LConn1
  Current Measurement/RConn1 -- A/RConn1
  Current Measurement1/RConn1 -- B/RConn1
  C/RConn1 -- Current Measurement2/RConn1
  Controlled Voltage Source/RConn1 -- Activation Switches/LConn1
  Activation Switches/LConn3 -- Controlled Voltage Source1/LConn1

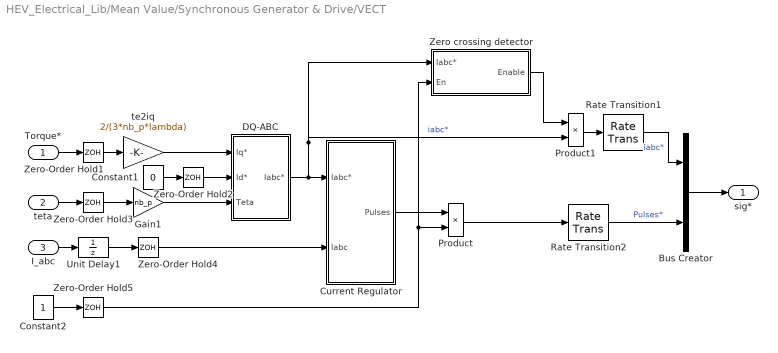
== system HEV_Electrical_Lib/Mean Value/Synchronous Generator & Drive/VECT ==
  Torque* : Inport
  teta : Inport  Port=2
  I_abc : Inport  Port=3
  Bus Creator : BusCreator  Inputs=2
  Constant1 : Constant  Value=0
  Constant2 : Constant
  Current Regulator : Subsystem
  DQ-ABC : Subsystem
  Gain1 : Gain  Gain=nb_p  SaturateOnIntegerOverflow=on  OutDataTypeStr=Inherit: Same as input  ParamDataTypeStr=Inherit: Same as input
  Product : Product  RndMeth=Zero
  Product1 : Product  RndMeth=Zero
  Rate Transition1 : RateTransition
  Rate Transition2 : RateTransition
  Unit Delay1 : UnitDelay  SampleTime=Ts  HasFrameUpgradeWarning=on
  Zero crossing detector : Subsystem
  Zero-Order Hold{1..5} (5 alike) : ZeroOrderHold  SampleTime=Ts_vect
  te2iq : Gain  Gain=2/(3*nb_p*lambda)  SaturateOnIntegerOverflow=on  OutDataTypeStr=Inherit: Same as input  ParamDataTypeStr=Inherit: Same as input
  sig* : Outport  VectorParamsAs1DForOutWhenUnconnected=off
  wires:
  I_abc/1 -> Unit Delay1/1
  DQ-ABC/1(Iabc*) -> Current Regulator/1(Iabc*), Product1/2, Zero crossing detector/1(Iabc*)  "iabc*"
  Unit Delay1/1 -> Zero-Order Hold4/1
  Gain1/1 -> DQ-ABC/3(Teta)
  Constant1/1 -> Zero-Order Hold2/1
  Torque*/1 -> Zero-Order Hold1/1
  Zero-Order Hold3/1 -> Gain1/1
  teta/1 -> Zero-Order Hold3/1
  Zero-Order Hold1/1 -> te2iq/1
  Zero-Order Hold2/1 -> DQ-ABC/2("Id* ")
  te2iq/1 -> DQ-ABC/1("Iq* ")
  Bus Creator/1 -> sig*/1
  Rate Transition2/1 -> Bus Creator/2  "Pulses*"
  Rate Transition1/1 -> Bus Creator/1  "iabc*"
  Zero-Order Hold4/1 -> Current Regulator/2(Iabc)
  Current Regulator/1(Pulses) -> Product/1
  Product/1 -> Rate Transition2/1
  Product1/1 -> Rate Transition1/1
  Constant2/1 -> Zero-Order Hold5/1
  Zero crossing detector/1(Enable) -> Product1/1
  Zero-Order Hold5/1 -> Product/2, Zero crossing detector/2(En)

== system HEV_Electrical_Lib/Mean Value/Synchronous Motor & Drive/GF ==
  In1 : Inport
  Out1 : Outport  VectorParamsAs1DForOutWhenUnconnected=off
  tag scope: Mot_TReq_SYS=global
  wires:
  In1/1 -> [Mot_TReq_SYS], Out1/1

== system HEV_Electrical_Lib/Mean Value/Synchronous Motor & Drive/Mux ==
  sig* : Inport
  m : Inport  Port=2
  Bus Creator : BusCreator  Inputs=2
  Ctrl : Outport  VectorParamsAs1DForOutWhenUnconnected=off
  wires:
  m/1 -> Bus Creator/2  "m"
  sig*/1 -> Bus Creator/1  "Signals*"
  Bus Creator/1 -> Ctrl/1

== system HEV_Electrical_Lib/Mean Value/Synchronous Motor & Drive/Subsystem ==
  In1 : Inport
  "+ -> -1" : Gain  Gain=30/pi
  Bus Selector : BusSelector  OutputSignals=Stator current is_a (A),Rotor speed wm (rad/s),Electromagnetic torque Te (N*m)
  Mux1 : Mux  Inputs=2
  Mux2 : Mux  Inputs=3
  Motor : Outport  VectorParamsAs1DForOutWhenUnconnected=off
  tag scope: MotorDrive=global
  wires:
  Mux2/1 -> [MotorDrive]
  Bus Selector/1 -> Mux2/1  "<Stator current is_a (A)>"
  Mux1/1 -> Mux2/3
  Bus Selector/3 -> Mux1/1  "<Electromagnetic torque Te (N*m)>"
  Bus Selector/2 -> "+ -> -1"/1  "<Rotor speed wm (rad/s)>"
  [Mot_TReq_SYS] -> Mux1/2
  "+ -> -1"/1 -> Mux2/2
  In1/1 -> Motor/1, Bus Selector/1

== system HEV_Electrical_Lib/Mean Value/Synchronous Motor & Drive/Subsystem1 ==
  Sig : Inport
  Bus Selector : BusSelector  OutputSignals=Electromagnetic torque Te (N*m)
  Ideal Rotational Motion Sensor : fl_lib/Mechanical/Mechanical Sensors/Ideal Rotational Motion Sensor  offset=0 rad
  Ideal Torque Source : fl_lib/Mechanical/Mechanical Sources/Ideal Torque Source
  Mechanical Rotational Reference : fl_lib/Mechanical/Rotational Elements/Mechanical Rotational Reference
  Mechanical Rotational Reference1 : fl_lib/Mechanical/Rotational Elements/Mechanical Rotational Reference
  PS-Simulink Converter : nesl_utility/PS-Simulink Converter  PhysicalDomain=network_engine_domain  SubClassName=ps_output  LeftPortType=input  RightPortType=output  PseudoPeriodic=off  Frequencies=[]  Unit=rad/s  AffineConversion=off
  Simulink-PS Converter : nesl_utility/Simulink-PS Converter  PhysicalDomain=network_engine_domain  SubClassName=ps_input  LeftPortType=input  RightPortType=output  PseudoPeriodic=off  Frequencies=[]  NoiseDistribution=none  NoiseParameters=[]  Unit=1  AffineConversion=off  FilteringAndDerivatives=zero  SimscapeFilterOrder=1  InputFilterTimeConstant=0.005  UdotUserProvided=0
  Sh : PMIOPort  Side=Right
  Spd : Outport  VectorParamsAs1DForOutWhenUnconnected=off
  wires:
  Bus Selector/1 -> Simulink-PS Converter/1  "<Electromagnetic torque Te (N*m)>"
  Sig/1 -> Bus Selector/1
  PS-Simulink Converter/1 -> Spd/1
  connections:
  Mechanical Rotational Reference/LConn1 -- Ideal Rotational Motion Sensor/RConn1
  Mechanical Rotational Reference1/LConn1 -- Ideal Torque Source/RConn2
  Ideal Torque Source/LConn1 -- Sh/RConn1 -- Ideal Rotational Motion Sensor/LConn1
  PS-Simulink Converter/LConn1 -- Ideal Rotational Motion Sensor/RConn2
  Simulink-PS Converter/RConn1 -- Ideal Torque Source/RConn1

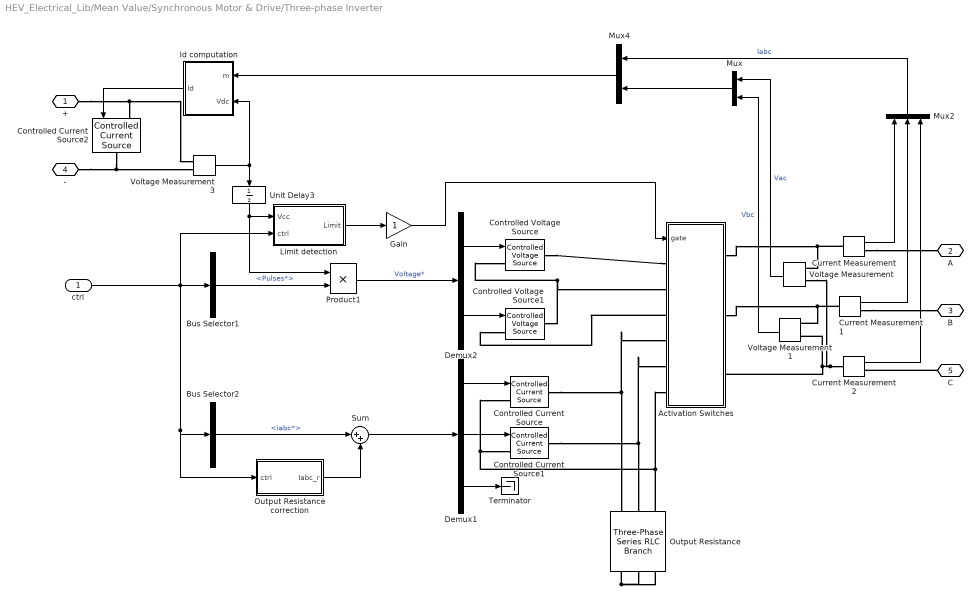
== system HEV_Electrical_Lib/Mean Value/Synchronous Motor & Drive/Three-phase Inverter ==
  ctrl : Inport
  Activation Switches : Subsystem
  Bus Selector1 : BusSelector  OutputSignals=Signals*.Pulses*
  Bus Selector2 : BusSelector  OutputSignals=Signals*.iabc*
  Controlled Current Source : powerlib/Electrical Sources/Controlled Current Source  Initialize=on  Source_Type=AC  Amplitude=0  Phase=0  Frequency=0  Measurements=None
      settings: SourceProductName=Simscape Electrical
  Controlled Current Source1 : powerlib/Electrical Sources/Controlled Current Source  Initialize=on  Source_Type=AC  Amplitude=0  Phase=0  Frequency=0  Measurements=None
      settings: SourceProductName=Simscape Electrical
  Controlled Current Source2 : powerlib/Electrical Sources/Controlled Current Source  Initialize=on  Source_Type=AC  Amplitude=0  Phase=0  Frequency=0  Measurements=None
      settings: SourceProductName=Simscape Electrical
  Controlled Voltage Source : powerlib/Electrical Sources/Controlled Voltage Source  Initialize=on  Source_Type=AC  Amplitude=0  Phase=0  Frequency=0  Measurements=None
      settings: SourceProductName=Simscape Electrical
  Controlled Voltage Source1 : powerlib/Electrical Sources/Controlled Voltage Source  Initialize=on  Source_Type=AC  Amplitude=0  Phase=0  Frequency=0  Measurements=None
      settings: SourceProductName=Simscape Electrical
  Current Measurement : powerlib/Measurements/Current Measurement  PhasorSimulation=off  OutputType=Complex  PSBequivalent=0
      settings: SourceProductName=Simscape Electrical
  Current Measurement1 : powerlib/Measurements/Current Measurement  PhasorSimulation=off  OutputType=Complex  PSBequivalent=0
      settings: SourceProductName=Simscape Electrical
  Current Measurement2 : powerlib/Measurements/Current Measurement  PhasorSimulation=off  OutputType=Complex  PSBequivalent=0
      settings: SourceProductName=Simscape Electrical
  Demux1 : Demux  Outputs=3
  Demux2 : Demux  Outputs=2
  Gain : Gain
  Id computation : Subsystem
  Limit detection : Subsystem
  Mux : Mux  Inputs=2
  Mux2 : Mux  Inputs=3
  Mux4 : Mux  Inputs=2
  Output Resistance : powerlib/Elements/Three-Phase Series RLC Branch  LConnTagsString=A|B|C  RConnTagsString=A|B|C  BranchType=R  Resistance=100*Resistance  Inductance=1e-3  Capacitance=1e-6  Measurements=Branch voltages and currents
      settings: SourceProductName=Simscape Electrical
  Output Resistance correction : Subsystem
  Product1 : Product  RndMeth=Zero
  Sum : Sum  Inputs=|++
  Terminator : Terminator
  Unit Delay3 : UnitDelay  SampleTime=Ts  HasFrameUpgradeWarning=on
  Voltage Measurement : powerlib/Measurements/Voltage Measurement  PhasorSimulation=off  OutputType=Complex  PSBequivalent=0
      settings: SourceProductName=Simscape Electrical
  Voltage Measurement1 : powerlib/Measurements/Voltage Measurement  PhasorSimulation=off  OutputType=Complex  PSBequivalent=0
      settings: SourceProductName=Simscape Electrical
  Voltage Measurement3 : powerlib/Measurements/Voltage Measurement  PhasorSimulation=off  OutputType=Complex  PSBequivalent=0
      settings: SourceProductName=Simscape Electrical
  + : PMIOPort  Side=Right
  A : PMIOPort  Port=2  Side=Left
  B : PMIOPort  Port=3  Side=Left
  - : PMIOPort  Port=4  Side=Right
  C : PMIOPort  Port=5  Side=Left
  wires:
  Output Resistance correction/1("Iabc_r ") -> Sum/2
  Id computation/1(Id) -> Controlled Current Source2/1
  Gain/1 -> Activation Switches/1(gate)
  Product1/1 -> Demux2/1  "Voltage*"
  ctrl/1 -> Output Resistance correction/1(ctrl), Bus Selector2/1, Limit detection/2(ctrl), Bus Selector1/1
  Unit Delay3/1 -> Limit detection/1(Vcc), Product1/1
  Sum/1 -> Demux1/1
  Limit detection/1(Limit) -> Gain/1
  Bus Selector2/1 -> Sum/1  "<iabc*>"
  Demux2/1 -> Controlled Voltage Source/1
  Demux2/2 -> Controlled Voltage Source1/1
  Demux1/3 -> Terminator/1
  Demux1/2 -> Controlled Current Source1/1
  Demux1/1 -> Controlled Current Source/1
  Bus Selector1/1 -> Product1/2  "<Pulses*>"
  Voltage Measurement3/1 -> Id computation/2(Vdc), Unit Delay3/1
  Mux2/1 -> Mux4/1  "Iabc"
  Mux4/1 -> Id computation/1(m)
  Current Measurement2/1 -> Mux2/3
  Mux/1 -> Mux4/2
  Voltage Measurement1/1 -> Mux/2  "Vbc"
  Voltage Measurement/1 -> Mux/1  "Vac"
  Current Measurement1/1 -> Mux2/2
  Current Measurement/1 -> Mux2/1
  connections:
  Activation Switches/LConn3 -- Controlled Voltage Source1/LConn1
  Controlled Voltage Source/RConn1 -- Activation Switches/LConn1
  C/RConn1 -- Current Measurement2/RConn1
  Current Measurement1/RConn1 -- B/RConn1
  Current Measurement/RConn1 -- A/RConn1
  Current Measurement1/LConn1 -- Activation Switches/RConn2 -- Voltage Measurement1/LConn1
  Controlled Voltage Source1/RConn1 -- Activation Switches/LConn2 -- Controlled Voltage Source/LConn1
  Current Measurement2/LConn1 -- Voltage Measurement1/LConn2 -- Activation Switches/RConn3 -- Voltage Measurement/LConn2
  Controlled Current Source1/RConn1 -- Activation Switches/LConn5 -- Output Resistance/LConn2
  Controlled Current Source/RConn1 -- Activation Switches/LConn4 -- Output Resistance/LConn1
  Current Measurement/LConn1 -- Activation Switches/RConn1 -- Voltage Measurement/LConn1
  Output Resistance/RConn1 -- Output Resistance/RConn2 -- Output Resistance/RConn3
  Output Resistance/LConn3 -- Controlled Current Source1/LConn1 -- Controlled Current Source/LConn1 -- Activation Switches/LConn6
  -/RConn1 -- Controlled Current Source2/RConn1 -- Voltage Measurement3/LConn2
  +/RConn1 -- Controlled Current Source2/LConn1 -- Voltage Measurement3/LConn1

== system HEV_Electrical_Lib/Mean Value/Synchronous Motor & Drive/Torque limitation ==
  N rad/s : Inport
  Torque : Inport  Port=2
  Abs1 : Abs  SaturateOnIntegerOverflow=on
  Gain : Gain  Gain=-1
  Saturation Dynamic : simulink/Discontinuities/Saturation Dynamic  OutMin=[]  OutMax=[]  OutDataTypeStr=Inherit: Same as second input  OutDataType=sfix(16)  OutScaling=2^-10  DoSatur=off
  Torque vs speed profile : Lookup  InputValues=HEV_Param.Motor.TorqSpdLUT.SpeedRPM*pi/30  Table=HEV_Param.Motor.TorqSpdLUT.TorqueNm
  torque : Outport  VectorParamsAs1DForOutWhenUnconnected=off
  wires:
  Gain/1 -> Saturation Dynamic/3
  Torque/1 -> Saturation Dynamic/2
  Saturation Dynamic/1 -> torque/1
  Torque vs speed profile/1 -> Gain/1, Saturation Dynamic/1
  Abs1/1 -> Torque vs speed profile/1
  N rad/s/1 -> Abs1/1
